simulink library "MoDesA_lib"  (R2017a)
settings: Solver=VariableStepAuto  StartTime=0.0  StopTime=10.0  RelTol=1e-3
libraries: MoDesA_lib x1
settings Model: Creator=streit  LastModifiedBy=streit

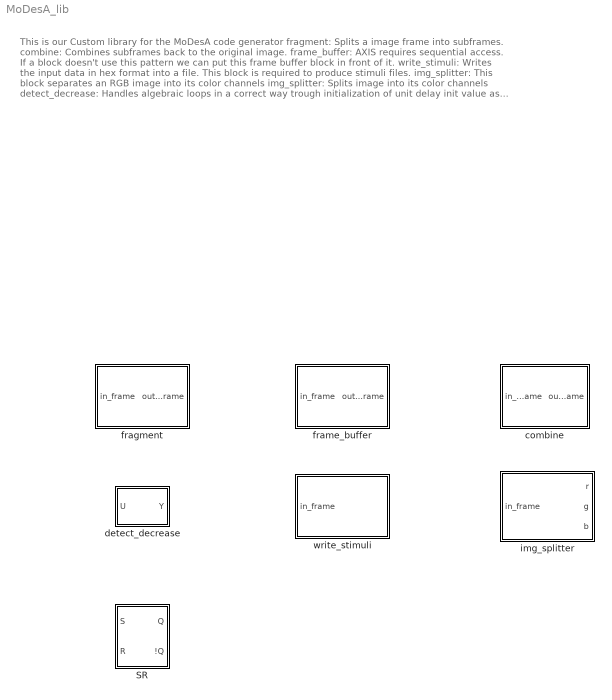
== system MoDesA_lib ==
  note: This is our Custom library for the MoDesA code generator
      | fragment: Splits a image frame into subframes.
      | combine: Combines subframes back to the original image.
      | frame_buffer: AXIS requires sequential access. If a block doesn't use this pattern we can put this frame buffer block in front of it.
      | write_stimuli: Writes the input data in hex format into a file. This block is required to produce stimuli files.
      | img_splitter: This block separates an RGB image into its color channels
      | img_splitter: Splits image into its color channels
      | detect_decrease: Handles algebraic loops in a correct way trough initialization of unit delay init value as Storage Class with ExportedGlobal attribute
      | SR: Handles algebraic loops in a correct way trough initialization of memory init value as Storage Class with ExportedGlobal attribute
  "SR " : Subsystem  mask(SRFlipFlop){initial_condition=0, StateIdentifier=initStateName}
      mask prompts: initial_condition "SimulinkBlocks:simulink_extras:InitialConditionstateOfQ_MP"; StateIdentifier "Simulink:blkprm_prompts:StateName"
      mask help: SimulinkBlocks:simulink_extras:SRFlipFlop_MD
      mask Help: web([docroot '/simulink/ref_extras/srflipflop.html'])
      mask TypeOptions StateIdentifier: Memory/StateIdentifier
  combine : Subsystem  mask(Combine){mask_d=50, image_size=[1200 1920], output_size=0}
      mask prompts: mask_d "Mask size"; image_size "Output image size"
      mask help: Combines fragments into an image of the specified size. Output image size and mask size must be equivalent to the corresponding Fragment block.
      mask init:
      | if size(image_size,2) == 2
      |     output_size = [image_size(1) image_size(2)];
      | else 
      |     output_size = [image_size(1) image_size(2) image_size(3)];
      | end
      mask Help: Enter the the size of the biggest mask and the size of the output image [height width (dim)]. The value of dim must be greater than 1, if specified. Values must be set according the corresponding Fragment Block.
      mask Display: text(0.5, 0.5, 'Combine', 'horizontalAlignment', 'center')
  detect_decrease : Subsystem  mask(Detect Decrease){vinit=0.0, InputProcessing=Columns as channels (frame based), OutDataTypeStr=boolean, StateName=initname}
      mask prompts: vinit "Simulink:masks:InitialCondition_MP"; InputProcessing "Input processing:"; OutDataTypeStr "Output data type"; StateName "Simulink:blkprm_prompts:StateName"
      mask help: Simulink:masks:DetectDecrease_MD
      mask init:
      | initDetectBlocks();
      mask TypeOptions InputProcessing: Simulink:masks:ColumnsAsChannelsFrameBased | Simulink:masks:ElementsAsChannelsSampleBased | Simulink:masks:Inherited
      mask TypeOptions OutDataTypeStr: Simulink:masks:uint8 | Simulink:masks:boolean
      mask TypeOptions StateName: Delay Input1/StateName
      mask Display: fprintf('U < U/z')
  fragment : Subsystem  mask(Fragmentation){mask_d=50, block_size=[40 40], out_size=0, image=0}
      mask prompts: mask_d "Mask size"; block_size "Block size"
      mask help: Fragments an input image in fragments of the specified block size. Mask size and block dimensions must be equivalent to the corresponding Combine block
      mask init:
      | if size(block_size,2) == 2
      |     out_size = [block_size(1)+mask_d block_size(2)+mask_d];
      | else 
      |     out_size = [block_size(1)+mask_d block_size(2)+mask_d block_size(3)];
      | end
      mask Help: Enter the the size of the biggest mask and the size of the fragments [height width (dim)]. The value of dim must be greater than 1, if specified. Values must be set according to the corresponding Combine Block.
      mask Display: text(0.5, 0.5, 'Fragment', 'horizontalAlignment', 'center')
  frame_buffer : Subsystem  mask(Frame Buffer){}
      mask help: Creates a buffer for one frame
      mask Help: Creates a buffer for one frame
      mask Display: text(0.5, 0.5, 'Frame Buffer', 'horizontalAlignment', 'center')
  img_splitter : Subsystem  Tag=hw_ip  mask(Image Split){}
      mask help: This Blocks splits an 3D image into its RGB components
      mask Help: This Blocks splits an 3D image into its RGB components
  write_stimuli : Subsystem  mask(writeStimuli){bound=1, instance=0}
      mask prompts: bound "Number of Stimuli"; instance "Instance Number"
      mask help: Creates the specified number of stimuli files from the input data per instance.
      mask init:
      | bound >= 0;
      | instance >= 0;
      mask Help:
      | Enter the number of stimuli files to be created.
      | If you use multiple write_stimuli blocks in the model, specify instance to distinguish between blocks.
      mask Display: text(0.5, 0.5, 'Stimuli', 'horizontalAlignment', 'center')

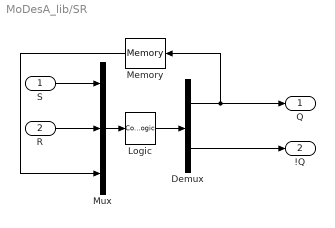
== system MoDesA_lib/SR  ==
  S : Inport
  R : Inport  Port=2
  Demux : Demux  Outputs=2
  Logic : CombinatorialLogic  TruthTable=[0 1;1 0;0 1;0 1;1 0;1 0;0 0;0 0]
  Memory : Memory  X0=initial_condition  InheritSampleTime=on  StateIdentifier=initStateName
  Mux : Mux  Inputs=3
  Q : Outport
  !Q : Outport  Port=2
  wires:
  R/1 -> Mux/2
  S/1 -> Mux/1
  Logic/1 -> Demux/1
  Memory/1 -> Mux/3
  Mux/1 -> Logic/1
  Demux/1 -> Q/1, Memory/1
  Demux/2 -> !Q/1

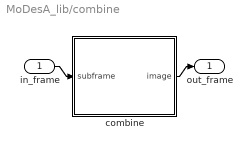
== system MoDesA_lib/combine ==
  in_frame : Inport
  "combine " : MATLAB Function  TreatAsAtomicUnit=on
  out_frame : Outport
  wires:
  "combine "/1(image) -> out_frame/1
  in_frame/1 -> "combine "/1(subframe)

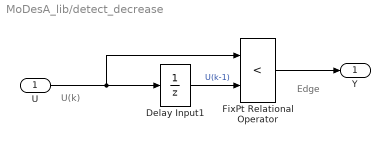
== system MoDesA_lib/detect_decrease ==
  note: U(k)
  note: Edge
  U : Inport
  Delay Input1 : UnitDelay  Description=Store in Global RAM  DisableCoverage=on  InitialCondition=vinit  InputProcessing=Columns as channels (frame based)  SampleTime=-1  StateName=initname
  FixPt Relational Operator : RelationalOperator  Operator=<  OutDataTypeStr=boolean  ZeroCross=off  RndMeth=Nearest
  Y : Outport
  wires:
  U/1 -> Delay Input1/1, FixPt Relational Operator/1
  FixPt Relational Operator/1 -> Y/1
  Delay Input1/1 -> FixPt Relational Operator/2  "U(k-1)"

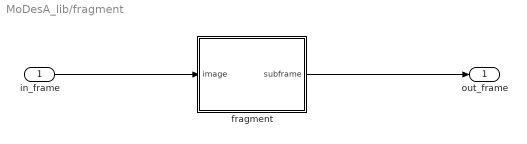
== system MoDesA_lib/fragment ==
  in_frame : Inport
  "fragment " : MATLAB Function  TreatAsAtomicUnit=on
  out_frame : Outport
  wires:
  "fragment "/1(subframe) -> out_frame/1
  in_frame/1 -> "fragment "/1(image)

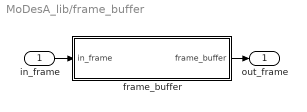
== system MoDesA_lib/frame_buffer ==
  in_frame : Inport
  "frame_buffer " : MATLAB Function  TreatAsAtomicUnit=on
  out_frame : Outport
  wires:
  in_frame/1 -> "frame_buffer "/1(in_frame)
  "frame_buffer "/1(frame_buffer) -> out_frame/1

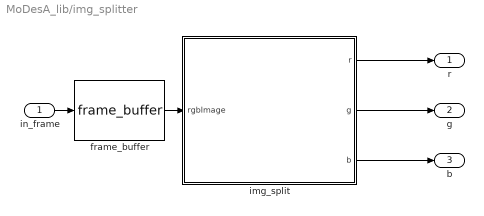
== system MoDesA_lib/img_splitter ==
  in_frame : Inport
  frame_buffer : MoDesA_lib/frame_buffer
      settings: SourceProductName=Custom Lib for MoDesA code generator
  img_split : MATLAB Function  TreatAsAtomicUnit=on
  r : Outport
  g : Outport  Port=2
  b : Outport  Port=3
  wires:
  img_split/3(b) -> b/1
  in_frame/1 -> frame_buffer/1
  img_split/1(r) -> r/1
  img_split/2(g) -> g/1
  frame_buffer/1 -> img_split/1(rgbImage)

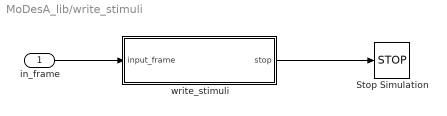
== system MoDesA_lib/write_stimuli ==
  in_frame : Inport
  Stop Simulation : Stop
  write_stimuli : MATLAB Function  TreatAsAtomicUnit=on
  wires:
  in_frame/1 -> write_stimuli/1(input_frame)
  write_stimuli/1(stop) -> Stop Simulation/1

== matlab function MoDesA_lib/frame_buffer/frame_buffer  ==
  data: in_frame input; frame_buffer output
%%
%--------------------------------------------------------------------------
% Copyright (c) 2017 Hardware-Software-Co-Design, Friedrich-
% Alexander-Universitaet Erlangen-Nuernberg (FAU), Germany.
% All rights reserved.
%
%
% This code and any associated documentation is provided "as is"
%
% IN NO EVENT SHALL HARDWARE-SOFTWARE-CO-DESIGN, FRIEDRICH-ALEXANDER-
% UNIVERSITAET ERLANGEN-NUERNBERG (FAU) BE LIABLE TO ANY PARTY FOR DIRECT,
% INDIRECT, SPECIAL, INCIDENTAL, OR CONSEQUENTIAL DAMAGES ARISING OUT
% OF THE USE OF THIS CODE AND ITS DOCUMENTATION, EVEN IF HARDWARE-
% SOFTWARE-CO-DESIGN, FRIEDRICH-ALEXANDER-UNIVERSITAET ERLANGEN-NUERNBERG
% (FAU) HAS BEEN ADVISED OF THE POSSIBILITY OF SUCH DAMAGE. THE
% AFOREMENTIONED EXCLUSIONS OF LIABILITY DO NOT APPLY IN CASE OF INTENT
% BY HARDWARE-SOFTWARE-CO-DESIGN, FRIEDRICH-ALEXANDER-UNIVERSITAET
% ERLANGEN-NUERNBERG (FAU).
%
% HARDWARE-SOFTWARE-CO-DESIGN, FRIEDRICH-ALEXANDER-UNIVERSITAET ERLANGEN-
% NUERNBERG (FAU), SPECIFICALLY DISCLAIMS ANY WARRANTIES, INCLUDING, BUT
% NOT LIMITED TO, THE IMPLIED WARRANTIES OF MERCHANTABILITY AND FITNESS
% FOR A PARTICULAR PURPOSE.
%
% THE CODE PROVIDED HEREUNDER IS ON AN "AS IS" BASIS, AND HARDWARE-
% SOFTWARE-CO-DESIGN, FRIEDRICH-ALEXANDER-UNIVERSITAET ERLANGEN-
% NUERNBERG (FAU) HAS NO OBLIGATION TO PROVIDE MAINTENANCE, SUPPORT,
% UPDATES, ENHANCEMENTS, OR MODIFICATIONS.
% -------------------------------------------------------------------------
%
%  @author Streit Franz-Josef 
%  @date   23 April 2018
%  @version 0.1
%  @brief This function creates memory in HW for non sequentiell access by 
%         the AXI-Stream interface
%
%
%%

function frame_buffer = frame_buffer(in_frame)
%#codegen
coder.inline('always')
tmp=cast(zeros(size(in_frame)),class(in_frame));

for i=1:numel(in_frame)
        tmp(i) = in_frame(i);
end
    frame_buffer = tmp;
end

== matlab function MoDesA_lib/img_splitter/img_split ==
  data: rgbImage input; r output; g output; b output
function [r,g,b] = img_split(rgbImage)
%#codegen
r = rgbImage(:,:,1); % Red channel
g = rgbImage(:,:,2); % Green channel
b = rgbImage(:,:,3); % Blue channel
end

== matlab function MoDesA_lib/write_stimuli/write_stimuli ==
  data: input_frame input; stop output; bound parameter; instance parameter
%%
%--------------------------------------------------------------------------
% Copyright (c) 2017 Hardware-Software-Co-Design, Friedrich-
% Alexander-Universitaet Erlangen-Nuernberg (FAU), Germany.
% All rights reserved.
%
%
% This code and any associated documentation is provided "as is"
%
% IN NO EVENT SHALL HARDWARE-SOFTWARE-CO-DESIGN, FRIEDRICH-ALEXANDER-
% UNIVERSITAET ERLANGEN-NUERNBERG (FAU) BE LIABLE TO ANY PARTY FOR DIRECT,
% INDIRECT, SPECIAL, INCIDENTAL, OR CONSEQUENTIAL DAMAGES ARISING OUT
% OF THE USE OF THIS CODE AND ITS DOCUMENTATION, EVEN IF HARDWARE-
% SOFTWARE-CO-DESIGN, FRIEDRICH-ALEXANDER-UNIVERSITAET ERLANGEN-NUERNBERG
% (FAU) HAS BEEN ADVISED OF THE POSSIBILITY OF SUCH DAMAGE. THE
% AFOREMENTIONED EXCLUSIONS OF LIABILITY DO NOT APPLY IN CASE OF INTENT
% BY HARDWARE-SOFTWARE-CO-DESIGN, FRIEDRICH-ALEXANDER-UNIVERSITAET
% ERLANGEN-NUERNBERG (FAU).
%
% HARDWARE-SOFTWARE-CO-DESIGN, FRIEDRICH-ALEXANDER-UNIVERSITAET ERLANGEN-
% NUERNBERG (FAU), SPECIFICALLY DISCLAIMS ANY WARRANTIES, INCLUDING, BUT
% NOT LIMITED TO, THE IMPLIED WARRANTIES OF MERCHANTABILITY AND FITNESS
% FOR A PARTICULAR PURPOSE.
%
% THE CODE PROVIDED HEREUNDER IS ON AN "AS IS" BASIS, AND HARDWARE-
% SOFTWARE-CO-DESIGN, FRIEDRICH-ALEXANDER-UNIVERSITAET ERLANGEN-
% NUERNBERG (FAU) HAS NO OBLIGATION TO PROVIDE MAINTENANCE, SUPPORT,
% UPDATES, ENHANCEMENTS, OR MODIFICATIONS.
% -------------------------------------------------------------------------
%
%  @author Streit Franz-Josef
%  @date   23 April 2018
%  @version 0.1
%  @brief This function transform the Simulink output data into rtl testbench
%         stimuli data
%
%
%%

function stop = write_stimuli(input_frame, bound, instance)

% validate input args
narginchk(1,Inf);

coder.extrinsic('fprintf')
coder.extrinsic('fopen')
coder.extrinsic('num2str')
coder.extrinsic('exist')
coder.extrinsic('mkdir')
coder.extrinsic('num2cell')
coder.extrinsic('numel')
persistent frame_cnt;

if isempty(frame_cnt)
    frame_cnt = 0;
end

% create stimuli folderbla
if (~isequal(exist('stimuli','dir'),7))
    mkdir 'stimuli';
end

% init this values to zero to let matlab know the size of the variable
% if not initialized it will produce the following error
% Colon operands must be all the same type, or mixed with real scalar doubles.
hex_value_size = 0;

if frame_cnt < bound
    stop = 0;
    %if we have no stimuli folder yet, create one
    if (~isequal(exist(['stimuli/input' instance],'dir'),7))
        mkdir(['stimuli/input' num2str(instance)]);
    end
    filename = ['stimuli/input' num2str(instance) '/' num2str(frame_cnt) '.hex'];
    [fileID, ~] = fopen(filename ,'w');
    switch class(input_frame)
        case 'double'
            % converts input data into hex values for rtl testbench stimuli
            hex_value = dec2hex(typecast(input_frame(:),'uint64'));
            hex_value_size = size(hex_value,1);
            for k = 1:hex_value_size
                fprintf(fileID,'%c',hex_value(k,:));
                fprintf(fileID,'\n');
            end
        case 'single'
            % converts input data into hex values for rtl testbench stimuli
            hex_value = dec2hex(typecast(input_frame(:),'uint32'));
            hex_value_size = size(hex_value,1);
            for k = 1:hex_value_size
                fprintf(fileID,'%c',hex_value(k,:));
                fprintf(fileID,'\n');
            end
        case 'int8'
            % converts input data into hex values for rtl testbench stimuli
            hex_value = dec2hex(typecast(input_frame(:),'uint8'));
            hex_values_size = size(hex_value,1);
            if hex_values_size == 1
                hex_value_size = numel(hex_value);
                printval = hex_value;
                for l = hex_value_size:(2-1)
                    printval = ['0' printval];
                end
                fprintf(fileID,'%c',printval);
                fprintf(fileID,'\n');
            else
                for k = 1:hex_values_size
                    hex_value_size = numel(hex_value(k,:));
                    printval = hex_value(k,:);
                    for l = hex_value_size:(2-1)
                        printval = ['0' printval];
                    end
                    fprintf(fileID,'%c',printval);
                    fprintf(fileID,'\n');
                end
            end
        case 'int16'
            % converts input data into hex values for rtl testbench stimuli
            hex_value = dec2hex(typecast(input_frame(:),'uint16'));
            hex_values_size = size(hex_value,1);
            if hex_values_size == 1
                hex_value_size = numel(hex_value);
                printval = hex_value;
                for l = hex_value_size:(4-1)
                    printval = ['0' printval];
                end
                fprintf(fileID,'%c',printval);
                fprintf(fileID,'\n');
            else
                for k = 1:hex_values_size
                    hex_value_size = numel(hex_value(k,:));
                    printval = hex_value(k,:);
                    for l = hex_value_size:(4-1)
                        printval = ['0' printval];
                    end
                    fprintf(fileID,'%c',printval);
                    fprintf(fileID,'\n');
                end
            end
        case 'int32'
            % converts input data into hex values for rtl testbench stimuli
            hex_value = dec2hex(typecast(input_frame(:),'uint32'));
            hex_values_size = size(hex_value,1);
            if hex_values_size == 1
                hex_value_size = numel(hex_value);
                printval = hex_value;
                for l = hex_value_size:(8-1)
                    printval = ['0' printval];
                end
                fprintf(fileID,'%c',printval);
                fprintf(fileID,'\n');
            else
                for k = 1:hex_values_size
                    hex_value_size = numel(hex_value(k,:));
                    printval = hex_value(k,:);
                    for l = hex_value_size:(8-1)
                        printval = ['0' printval];
                    end
                    fprintf(fileID,'%c',printval);
                    fprintf(fileID,'\n');
                end
            end
        case 'int64'
            % converts input data into hex values for rtl testbench stimuli
            hex_value = dec2hex(typecast(input_frame(:),'uint64'));
            hex_values_size = size(hex_value,1);
            if hex_values_size == 1
                hex_value_size = numel(hex_value);
                printval = hex_value;
                for l = hex_value_size:(16-1)
                    printval = ['0' printval];
                end
                fprintf(fileID,'%c',printval);
                fprintf(fileID,'\n');
            else
                for k = 1:hex_values_size
                    hex_value_size = numel(hex_value(k,:));
                    printval = hex_value(k,:);
                    for l = hex_value_size:(16-1)
                        printval = ['0' printval];
                    end
                    fprintf(fileID,'%c',printval);
                    fprintf(fileID,'\n');
                end
            end
        case 'uint8'
            % converts input data into hex values for rtl testbench stimuli
            hex_value = dec2hex(typecast(input_frame(:),'uint8'));
            hex_values_size = size(hex_value,1);
            if hex_values_size == 1
                hex_value_size = numel(hex_value);
                printval = hex_value;
                for l = hex_value_size:(2-1)
                    printval = ['0' printval];
                end
                fprintf(fileID,'%c',printval);
                fprintf(fileID,'\n');
            else
                for k = 1:hex_values_size
                    hex_value_size = numel(hex_value(k,:));
                    printval = hex_value(k,:);
                    for l = hex_value_size:(2-1)
                        printval = ['0' printval];
                    end
                    fprintf(fileID,'%c',printval);
                    fprintf(fileID,'\n');
                end
            end
        case 'uint16'
            % converts input data into hex values for rtl testbench stimuli
            hex_value = dec2hex(typecast(input_frame(:),'uint16'));
            hex_values_size = size(hex_value,1);
            if hex_values_size == 1
                hex_value_size = numel(hex_value);
                printval = hex_value;
                for l = hex_value_size:(4-1)
                    printval = ['0' printval];
                end
                fprintf(fileID,'%c',printval);
                fprintf(fileID,'\n');
            else
                for k = 1:hex_values_size
                    hex_value_size = numel(hex_value(k,:));
                    printval = hex_value(k,:);
                    for l = hex_value_size:(4-1)
                        printval = ['0' printval];
                    end
                    fprintf(fileID,'%c',printval);
                    fprintf(fileID,'\n');
                end
            end
        case 'uint32'
            % converts input data into hex values for rtl testbench stimuli
            hex_value = dec2hex(typecast(input_frame(:),'uint32'));
            hex_values_size = size(hex_value,1);
            if hex_values_size == 1
                hex_value_size = numel(hex_value);
                printval = hex_value;
                for l = hex_value_size:(8-1)
                    printval = ['0' printval];
                end
                fprintf(fileID,'%c',printval);
                fprintf(fileID,'\n');
            else
                for k = 1:hex_values_size
                    hex_value_size = numel(hex_value(k,:));
                    printval = hex_value(k,:);
                    for l = hex_value_size:(8-1)
                        printval = ['0' printval];
                    end
                    fprintf(fileID,'%c',printval);
                    fprintf(fileID,'\n');
                end
            end
        case 'uint64'
            % converts input data into hex values for rtl testbench stimuli
            hex_value = dec2hex(typecast(input_frame(:),'uint64'));
            hex_values_size = size(hex_value,1);
            if hex_values_size == 1
                hex_value_size = numel(hex_value);
                printval = hex_value;
                for l = hex_value_size:(16-1)
                    printval = ['0' printval];
                end
                fprintf(fileID,'%c',printval);
                fprintf(fileID,'\n');
            else
                for k = 1:hex_values_size
                    hex_value_size = numel(hex_value(k,:));
                    printval = hex_value(k,:);
                    for l = hex_value_size:(16-1)
                        printval = ['0' printval];
                    end
                    fprintf(fileID,'%c',printval);
                    fprintf(fileID,'\n');
                end
            end
        otherwise
            warning('MATLAB::write_stimuli.m Data Type %s not supported for stimuli file generation',class(input_frame))
    end
    fclose(fileID);
else
    stop = 1;
end
frame_cnt = frame_cnt+1;
end

== matlab function MoDesA_lib/fragment/fragment  ==
  data: subframe output uint8 size=out_size; image input; mask_d parameter uint16; block_size parameter
%%
%--------------------------------------------------------------------------
% Copyright (c) 2017 Hardware-Software-Co-Design, Friedrich-
% Alexander-Universitaet Erlangen-Nuernberg (FAU), Germany.
% All rights reserved.
%
%
% This code and any associated documentation is provided "as is"
%
% IN NO EVENT SHALL HARDWARE-SOFTWARE-CO-DESIGN, FRIEDRICH-ALEXANDER-
% UNIVERSITAET ERLANGEN-NUERNBERG (FAU) BE LIABLE TO ANY PARTY FOR DIRECT,
% INDIRECT, SPECIAL, INCIDENTAL, OR CONSEQUENTIAL DAMAGES ARISING OUT
% OF THE USE OF THIS CODE AND ITS DOCUMENTATION, EVEN IF HARDWARE-
% SOFTWARE-CO-DESIGN, FRIEDRICH-ALEXANDER-UNIVERSITAET ERLANGEN-NUERNBERG
% (FAU) HAS BEEN ADVISED OF THE POSSIBILITY OF SUCH DAMAGE. THE
% AFOREMENTIONED EXCLUSIONS OF LIABILITY DO NOT APPLY IN CASE OF INTENT
% BY HARDWARE-SOFTWARE-CO-DESIGN, FRIEDRICH-ALEXANDER-UNIVERSITAET
% ERLANGEN-NUERNBERG (FAU).
%
% HARDWARE-SOFTWARE-CO-DESIGN, FRIEDRICH-ALEXANDER-UNIVERSITAET ERLANGEN-
% NUERNBERG (FAU), SPECIFICALLY DISCLAIMS ANY WARRANTIES, INCLUDING, BUT
% NOT LIMITED TO, THE IMPLIED WARRANTIES OF MERCHANTABILITY AND FITNESS
% FOR A PARTICULAR PURPOSE.
%
% THE CODE PROVIDED HEREUNDER IS ON AN "AS IS" BASIS, AND HARDWARE-
% SOFTWARE-CO-DESIGN, FRIEDRICH-ALEXANDER-UNIVERSITAET ERLANGEN-
% NUERNBERG (FAU) HAS NO OBLIGATION TO PROVIDE MAINTENANCE, SUPPORT,
% UPDATES, ENHANCEMENTS, OR MODIFICATIONS.
% -------------------------------------------------------------------------
%
%  @author Streit Franz-Josef 
%  @date   23 April 2018
%  @version 0.1
%  @brief This function splits the original image into subframes depending
%         on your mask size and subframe size
%
%
%%
%image: Block input signal
%mask_d, block_size: Mask parameters
function subframe = fragment(image, mask_d, block_size)
%#codegen
persistent i;
persistent j;

dim = uint16(size(image));
rows = uint16(dim(1));
cols = uint16(dim(2));

if size(block_size,2) == 2
   ch = uint8(1);
else 
    ch = uint8(block_size(3));
end
        

%size of the biggest mask used in processing algorithm
%must be same as in combine
% mask_d = uint8(5); 

%dimensions of the used data without overlapping boundary
%must be same as in combine
block_a = uint16(block_size(2));
block_b = uint16(block_size(1));

assert(block_a>=mask_d && block_b>=mask_d);

%size of one subframe that is transferred
subframe_a = uint16(block_a + mask_d);
subframe_b = uint16(block_b + mask_d);

if(ch > 1)
    subframe = uint8(zeros(subframe_b, subframe_a,ch));
else
    subframe = uint8(zeros(subframe_b, subframe_a,1));
end

number_subframes_x = uint16(idivide(cols, block_a, 'ceil'));
number_subframes_y = uint16(idivide(rows, block_b, 'ceil'));

%padding for border handling, must be double for grayscale images
pad_x = double(mask_d +block_a - mod(cols, block_a));
pad_y = double(mask_d + block_b - mod(rows, block_b));
img_padded = uint8(padarray(image, [pad_y, pad_x], 'symmetric'));

if isempty(i)
    i = uint16(1);
    j = uint16(1);
else
    i = i + uint16(1);
    if number_subframes_x < i
        i = uint16(1);
        j = j + uint16(1) ;
    end
    if number_subframes_y < j
        j = uint16(1);
    end
end    

top_row =  uint16((j-1)*block_b+1 + pad_y-mask_d);
left_row =  uint16((i-1)*block_a+1 + pad_x-mask_d);

if(ch > 1)
    tmp = uint8(img_padded(top_row:top_row+subframe_b-1,left_row:left_row+subframe_a-1,1:ch));
    subframe = uint8(tmp(1:subframe_b, 1:subframe_a, 1:ch));
else
   tmp = uint8(img_padded(top_row:top_row+subframe_b-1,left_row:left_row+subframe_a-1,1));
   subframe = uint8(tmp(1:subframe_b, 1:subframe_a, 1)); 
end

end

== matlab function MoDesA_lib/combine/combine  ==
  data: subframe input; image output size=output_size; mask_d parameter; image_size parameter
%%
%--------------------------------------------------------------------------
% Copyright (c) 2017 Hardware-Software-Co-Design, Friedrich-
% Alexander-Universitaet Erlangen-Nuernberg (FAU), Germany.
% All rights reserved.
%
%
% This code and any associated documentation is provided "as is"
%
% IN NO EVENT SHALL HARDWARE-SOFTWARE-CO-DESIGN, FRIEDRICH-ALEXANDER-
% UNIVERSITAET ERLANGEN-NUERNBERG (FAU) BE LIABLE TO ANY PARTY FOR DIRECT,
% INDIRECT, SPECIAL, INCIDENTAL, OR CONSEQUENTIAL DAMAGES ARISING OUT
% OF THE USE OF THIS CODE AND ITS DOCUMENTATION, EVEN IF HARDWARE-
% SOFTWARE-CO-DESIGN, FRIEDRICH-ALEXANDER-UNIVERSITAET ERLANGEN-NUERNBERG
% (FAU) HAS BEEN ADVISED OF THE POSSIBILITY OF SUCH DAMAGE. THE
% AFOREMENTIONED EXCLUSIONS OF LIABILITY DO NOT APPLY IN CASE OF INTENT
% BY HARDWARE-SOFTWARE-CO-DESIGN, FRIEDRICH-ALEXANDER-UNIVERSITAET
% ERLANGEN-NUERNBERG (FAU).
%
% HARDWARE-SOFTWARE-CO-DESIGN, FRIEDRICH-ALEXANDER-UNIVERSITAET ERLANGEN-
% NUERNBERG (FAU), SPECIFICALLY DISCLAIMS ANY WARRANTIES, INCLUDING, BUT
% NOT LIMITED TO, THE IMPLIED WARRANTIES OF MERCHANTABILITY AND FITNESS
% FOR A PARTICULAR PURPOSE.
%
% THE CODE PROVIDED HEREUNDER IS ON AN "AS IS" BASIS, AND HARDWARE-
% SOFTWARE-CO-DESIGN, FRIEDRICH-ALEXANDER-UNIVERSITAET ERLANGEN-
% NUERNBERG (FAU) HAS NO OBLIGATION TO PROVIDE MAINTENANCE, SUPPORT,
% UPDATES, ENHANCEMENTS, OR MODIFICATIONS.
% -------------------------------------------------------------------------
%
%  @author Streit Franz-Josef 
%  @date   23 April 2018
%  @version 0.1
%  @brief This function combines the subframes into the original image
%   
%
%%

%subframe: Block input signal
%mask_d, image_size: Mask parameters
function image = combine(subframe, mask_d, image_size)
%#codegen
persistent img_padded;
persistent i;
persistent j;

% get the output image size
rows = uint16(image_size(1));
cols = uint16(image_size(2));

%calculate channels based on mask parameters
if size(image_size,2) == 2
   ch = uint8(1);
else 
    ch = uint8(image_size(3));
end

subframe_size = uint16(size(subframe));

%dimensions of the used data without overlapping boundary
%must be same as in fragment
block_a = uint16(subframe_size(2)-mask_d);
block_b = uint16(subframe_size(1)-mask_d);
assert(block_a>=mask_d && block_b>=mask_d);

%padding for border handling
pad_y = uint16(block_b - mod(rows, block_b));
pad_x = uint16(block_a - mod(cols, block_a));

number_subframes_x = uint16(idivide(cols, block_a, 'ceil'));
number_subframes_y = uint16(idivide(rows, block_b, 'ceil'));

if isempty(i)
    %initialize output white
    img_padded =  uint8(ones(rows+2*pad_y, cols+2*pad_x,ch)*255);
    i = uint16(1);
    j = uint16(1);
else
    i = i + 1;
    if number_subframes_x < i
        i = uint16(1);
        j = j + uint16(1);
    end
    if number_subframes_y < j
        j = uint16(1);
    end
end

top_row =  uint16((j-1)*block_b+1 + pad_y);
left_row =  uint16((i-1)*block_a+1 + pad_x);
img_padded(top_row:top_row+block_b-1,left_row:left_row+block_a-1,1:ch) = uint8(subframe(mask_d+1:mask_d+block_b, mask_d+1:mask_d+block_a,1:ch));
image = uint8(img_padded(pad_y+1:pad_y+rows, pad_x+1:pad_x+cols,1:ch));
